simulink model "mov_tras_simulink"  (R2024b)
settings: Solver=VariableStepAuto  StartTime=0.0  StopTime=10  RelTol=1e-3
InitFcn:
  | m1 = 290;     % kg
  | m2 = 59;      % kg
  | b1 = 1000;    % Ns/m
  | k1 = 16182;   % N/m
  | k2 = 19000;   % N/m
  | f = 0;        % N
settings Model: Creator=PC WHALE

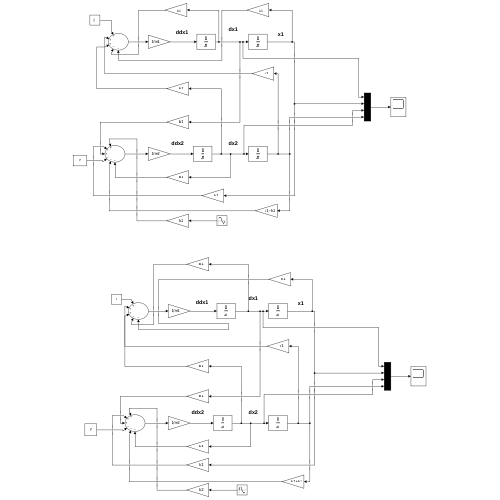
[thumbnail: Simulink's stored preview of the top-level diagram]
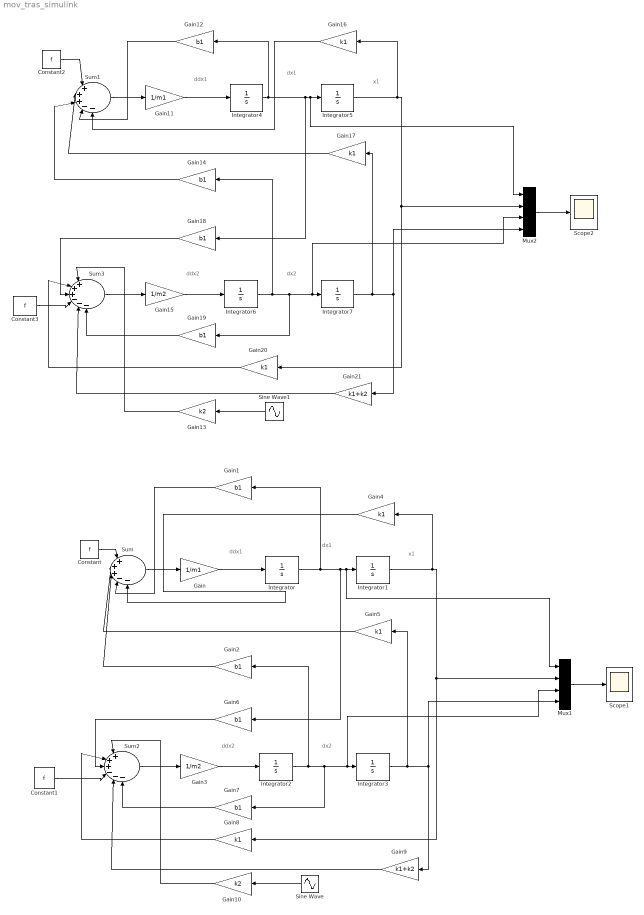
== system mov_tras_simulink ==
  note: ddx1
  note: dx1
  note: x1
  note: ddx2
  note: dx2
  note: ddx2
  note: x1
  note: dx2
  note: ddx1
  note: dx1
  Constant{,1..3} (4 alike) : Constant  Value=f
  Gain : Gain  Gain=1/m1
  Gain{1..2,6..7,12,14,18..19} (8 alike) : Gain  Gain=b1
  Gain10 : Gain  Gain=k2
  Gain11 : Gain  Gain=1/m1
  Gain13 : Gain  Gain=k2
  Gain15 : Gain  Gain=1/m2
  Gain{4..5,8,16..17,20} (6 alike) : Gain  Gain=k1
  Gain21 : Gain  Gain=k1+k2
  Gain3 : Gain  Gain=1/m2
  Gain9 : Gain  Gain=k1+k2
  Integrator{,1..7} (8 alike) : Integrator
  Mux1 : Mux
  Mux2 : Mux
  Scope1 : Scope
  Scope2 : Scope
  Sine Wave : Sin  Amplitude=0.05  Frequency=0.5*pi  SampleTime=0
  Sine Wave1 : Sin  Amplitude=0.05  Frequency=20*pi  SampleTime=0
  Sum : Sum  Inputs=|+++--
  Sum1 : Sum  Inputs=|+++--
  Sum2 : Sum  Inputs=|+++---
  Sum3 : Sum  Inputs=|+++---
  wires:
  Gain/1 -> Integrator/1
  Sum/1 -> Gain/1
  Integrator/1 -> Gain1/1, Mux1/1, Integrator1/1, Gain6/1
  Gain1/1 -> Sum/4
  Integrator1/1 -> Gain4/1, Mux1/2, Gain8/1
  Sum2/1 -> Gain3/1
  Integrator2/1 -> Gain7/1, Mux1/3, Integrator3/1, Gain2/1
  Gain3/1 -> Integrator2/1
  Gain2/1 -> Sum/3
  Gain4/1 -> Sum/5
  Integrator3/1 -> Gain5/1, Mux1/4, Gain9/1
  Gain5/1 -> Sum/2
  Constant/1 -> Sum/1
  Gain6/1 -> Sum2/3
  Gain7/1 -> Sum2/6
  Gain8/1 -> Sum2/2
  Gain9/1 -> Sum2/5
  Gain10/1 -> Sum2/1
  Constant1/1 -> Sum2/4
  Mux1/1 -> Scope1/1
  Sine Wave/1 -> Gain10/1
  Mux2/1 -> Scope2/1
  Gain13/1 -> Sum3/1
  Gain19/1 -> Sum3/6
  Sine Wave1/1 -> Gain13/1
  Gain21/1 -> Sum3/5
  Gain16/1 -> Sum1/5
  Integrator5/1 -> Gain16/1, Mux2/2, Gain20/1
  Integrator4/1 -> Mux2/1, Integrator5/1, Gain18/1, Gain12/1
  Gain14/1 -> Sum1/3
  Gain18/1 -> Sum3/3
  Gain20/1 -> Sum3/2
  Integrator7/1 -> Gain17/1, Mux2/4, Gain21/1
  Integrator6/1 -> Gain19/1, Mux2/3, Integrator7/1, Gain14/1
  Gain11/1 -> Integrator4/1
  Gain12/1 -> Sum1/4
  Sum3/1 -> Gain15/1
  Constant3/1 -> Sum3/4
  Sum1/1 -> Gain11/1
  Gain15/1 -> Integrator6/1
  Gain17/1 -> Sum1/2
  Constant2/1 -> Sum1/1
